simulink model "control_pos_no_lineal"  (R2020a)
settings: Solver=VariableStepAuto  StartTime=0.0  StopTime=5  RelTol=1e-3
values from neighbouring files (symbols this model uses):
  Kp = (2*pi*freq)^2*eye(2)    [init_control_cartesiano.m]
  Kv = 2*sqrt(Kp)*eye(2)    [init_control_cartesiano.m]
  Robot = Robot.perturb(0.8)    [init_control_cartesiano.m]
undefined symbols (not defined in the file or in its folder): coriolis
libraries: roblocks x16, simulink x2
settings Model: Creator=Gianfranco  LastModifiedBy=HP

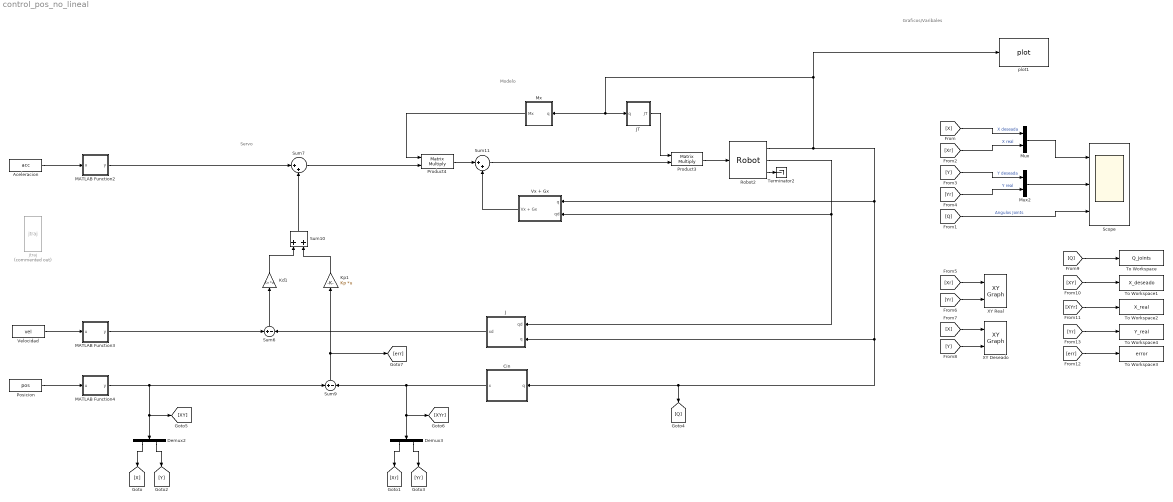
== system control_pos_no_lineal ==
  note: Graficos/Varibales
  note: Modelo
  note: Servo
  Aceleracion : FromWorkspace  VariableName=acc  SampleTime=-1  OutputAfterFinalValue=Holding final value
  Cin : Subsystem
  Demux2 : Demux  Outputs=2
  Demux3 : Demux  Outputs=2
  J : Subsystem
  JT : Subsystem
  Kd1 : Gain  Gain=Kv  Multiplication=Matrix(K*u)  SaturateOnIntegerOverflow=on  OutDataTypeStr=Inherit: Same as input  ParamDataTypeStr=Inherit: Same as input
  Kp1 : Gain  Gain=Kp  Multiplication=Matrix(K*u)  SaturateOnIntegerOverflow=on  OutDataTypeStr=Inherit: Same as input  ParamDataTypeStr=Inherit: Same as input
  MATLAB Function2 : MATLAB Function  TreatAsAtomicUnit=on
  MATLAB Function3 : MATLAB Function  TreatAsAtomicUnit=on
  MATLAB Function4 : MATLAB Function  TreatAsAtomicUnit=on
  Mux : Mux  Inputs=2
  Mux2 : Mux  Inputs=2
  Mx : Subsystem
  Posicion : FromWorkspace  VariableName=pos  SampleTime=-1  OutputAfterFinalValue=Holding final value
  Product3 : Product  Multiplication=Matrix(*)
  Product4 : Product  Multiplication=Matrix(*)
  Robot2 : roblocks/Arm/Robot  robot=Robot  q0=q0
      link override Integrator: InitialCondition=0
  Scope : Scope  NumInputPorts=3
  Sum10 : Sum  SaturateOnIntegerOverflow=on
  Sum11 : Sum  Inputs=|++  InputSameDT=on  SaturateOnIntegerOverflow=on  OutDataTypeStr=Inherit: Same as first input
  Sum6 : Sum  Inputs=+|-  InputSameDT=on  SaturateOnIntegerOverflow=on  OutDataTypeStr=Inherit: Same as first input
  Sum7 : Sum  Inputs=|++  InputSameDT=on  SaturateOnIntegerOverflow=on  OutDataTypeStr=Inherit: Same as first input
  Sum9 : Sum  Inputs=+|-  InputSameDT=on  SaturateOnIntegerOverflow=on  OutDataTypeStr=Inherit: Same as first input
  Terminator2 : Terminator
  To Workspace : ToWorkspace  VariableName=Q_joints  SaveFormat=Timeseries  SampleTime=-1
  To Workspace1 : ToWorkspace  VariableName=X_deseado  SaveFormat=Timeseries  SampleTime=-1
  To Workspace2 : ToWorkspace  VariableName=X_real  SaveFormat=Timeseries  SampleTime=-1
  To Workspace3 : ToWorkspace  VariableName=error  SaveFormat=Timeseries  SampleTime=-1
  To Workspace4 : ToWorkspace  VariableName=Y_real  SaveFormat=Timeseries  SampleTime=-1
  Velocidad : FromWorkspace  VariableName=vel  SampleTime=-1  OutputAfterFinalValue=Holding final value
  Vx + Gx : Subsystem
  XY Deseado : simulink/Sinks/XY Graph  xmin=-2  xmax=2  ymin=-2  ymax=2  st=-1
  XY Real : simulink/Sinks/XY Graph  xmin=-2  xmax=2  ymin=-2  ymax=2  st=-1
  jtraj : roblocks/Toolbox/jtraj  Commented=on  q0=[0 0 0 0 0 0]  qf=[pi/4 pi/2 -pi/2 0 0 0]  tmax=10  ts=0.02
  plot1 : roblocks/Arm/plot  robot=Robot  fps=30  holdplot=on
  wires:
  Posicion/1 -> MATLAB Function4/1(u)
  Product3/1 -> Robot2/1
  Sum7/1 -> Product4/2
  Sum6/1 -> Kd1/1
  Sum9/1 -> [err], Kp1/1
  Product4/1 -> Sum11/1
  Aceleracion/1 -> MATLAB Function2/1(u)
  Velocidad/1 -> MATLAB Function3/1(u)
  Kd1/1 -> Sum10/1
  Robot2/3 -> Terminator2/1
  Kp1/1 -> Sum10/2
  Sum10/1 -> Sum7/2
  Mx/1(Mx) -> Product4/1
  Sum11/1 -> Product3/2
  JT/1(JT) -> Product3/1
  Robot2/2 -> Vx + Gx/2(qd), J/1(qd)
  Robot2/1 -> [Q], Cin/1(q), J/2(q), Vx + Gx/1(q), JT/1(q), Mx/1(q), plot1/1
  MATLAB Function2/1(y) -> Sum7/1
  MATLAB Function3/1(y) -> Sum6/1
  Vx + Gx/1(Vx + Gx) -> Sum11/2
  J/1(xd) -> Sum6/2
  Mux/1 -> Scope/1
  Demux3/2 -> [Yr]
  Demux3/1 -> [Xr]
  [X] -> Mux/1  "X deseada"
  [Xr] -> Mux/2  "X real"
  [Y] -> Mux2/1  "Y deseada"
  [Yr] -> Mux2/2  "Y real"
  Mux2/1 -> Scope/2
  [Q] -> Scope/3  "Angulos Joints"
  [Xr] -> XY Real/1
  [Yr] -> XY Real/2
  [Y] -> XY Deseado/2
  [X] -> XY Deseado/1
  Cin/1(x) -> [XYr], Demux3/1, Sum9/2
  [XY] -> To Workspace1/1
  [Q] -> To Workspace/1
  [XYr] -> To Workspace2/1
  [err] -> To Workspace3/1
  Demux2/1 -> [X]
  Demux2/2 -> [Y]
  MATLAB Function4/1(y) -> Sum9/1, Demux2/1, [XY]
  [Yr] -> To Workspace4/1

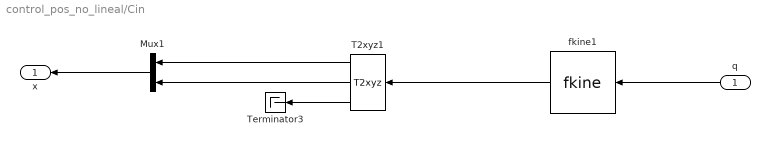
== system control_pos_no_lineal/Cin ==
  q : Inport
  Mux1 : Mux  Inputs=2
  T2xyz1 : roblocks/Toolbox/T2xyz
  Terminator3 : Terminator
  fkine1 : roblocks/Arm/fkine  robot=Robot
  x : Outport
  wires:
  T2xyz1/3 -> Terminator3/1
  fkine1/1 -> T2xyz1/1
  Mux1/1 -> x/1
  T2xyz1/2 -> Mux1/2
  T2xyz1/1 -> Mux1/1
  q/1 -> fkine1/1

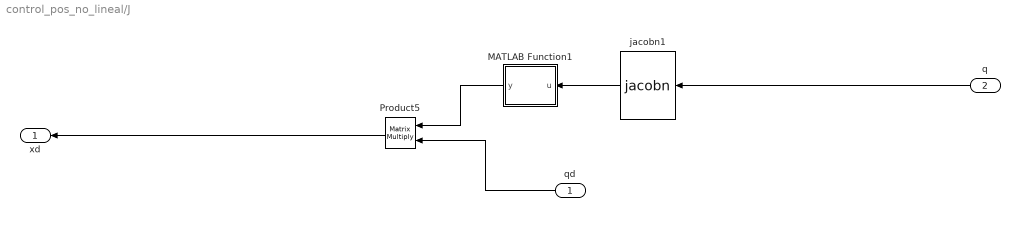
== system control_pos_no_lineal/J ==
  qd : Inport
  q : Inport  Port=2
  MATLAB Function1 : MATLAB Function  TreatAsAtomicUnit=on
  Product5 : Product  Multiplication=Matrix(*)
  jacobn1 : roblocks/Arm/jacobn  robot=Robot
  xd : Outport
  wires:
  jacobn1/1 -> MATLAB Function1/1(u)
  Product5/1 -> xd/1
  MATLAB Function1/1(y) -> Product5/1
  qd/1 -> Product5/2
  q/1 -> jacobn1/1

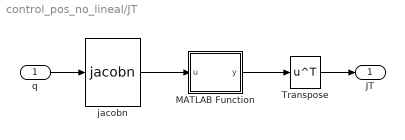
== system control_pos_no_lineal/JT ==
  q : Inport
  MATLAB Function : MATLAB Function  TreatAsAtomicUnit=on
  Transpose : Math  Operator=transpose  SaturateOnIntegerOverflow=on
  jacobn : roblocks/Arm/jacobn  robot=Robot
  JT : Outport
  wires:
  q/1 -> jacobn/1
  jacobn/1 -> MATLAB Function/1(u)
  Transpose/1 -> JT/1
  MATLAB Function/1(y) -> Transpose/1

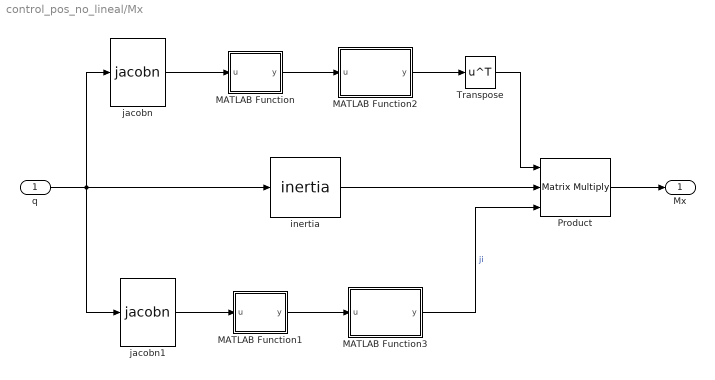
== system control_pos_no_lineal/Mx ==
  q : Inport
  MATLAB Function : MATLAB Function  TreatAsAtomicUnit=on
  MATLAB Function1 : MATLAB Function  TreatAsAtomicUnit=on
  MATLAB Function2 : MATLAB Function  TreatAsAtomicUnit=on
  MATLAB Function3 : MATLAB Function  TreatAsAtomicUnit=on
  Product : Product  Inputs=3  Multiplication=Matrix(*)
  Transpose : Math  Operator=transpose  SaturateOnIntegerOverflow=on
  inertia : roblocks/Arm/inertia  robot=Robot
  jacobn : roblocks/Arm/jacobn  robot=Robot
  jacobn1 : roblocks/Arm/jacobn  robot=Robot
  Mx : Outport
  wires:
  q/1 -> jacobn1/1, inertia/1, jacobn/1
  jacobn1/1 -> MATLAB Function1/1(u)
  MATLAB Function1/1(y) -> MATLAB Function3/1(u)
  Product/1 -> Mx/1
  inertia/1 -> Product/2
  jacobn/1 -> MATLAB Function/1(u)
  Transpose/1 -> Product/1
  MATLAB Function/1(y) -> MATLAB Function2/1(u)
  MATLAB Function3/1(y) -> Product/3  "ji"
  MATLAB Function2/1(y) -> Transpose/1

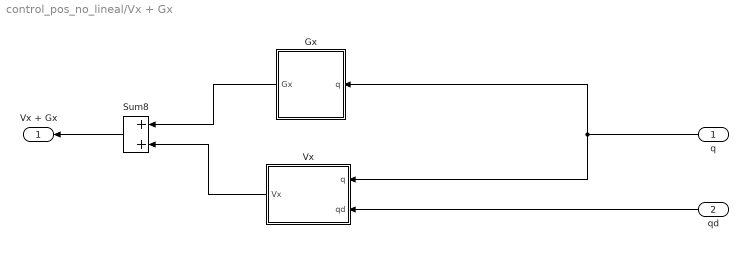
== system control_pos_no_lineal/Vx + Gx ==
  q : Inport
  qd : Inport  Port=2
  Gx : Subsystem
  Sum8 : Sum
  Vx : Subsystem
  Vx + Gx : Outport
  wires:
  Gx/1(Gx) -> Sum8/1
  Vx/1(Vx) -> Sum8/2
  Sum8/1 -> Vx + Gx/1
  qd/1 -> Vx/2(qd)
  q/1 -> Gx/1(q), Vx/1(q)

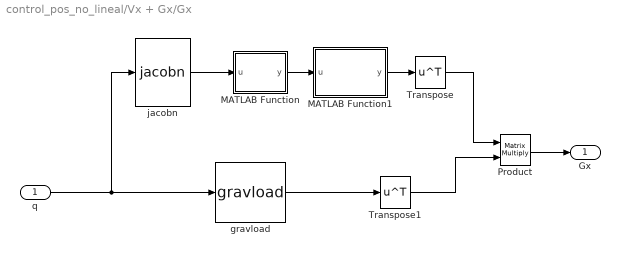
== system control_pos_no_lineal/Vx + Gx/Gx ==
  q : Inport
  MATLAB Function : MATLAB Function  TreatAsAtomicUnit=on
  MATLAB Function1 : MATLAB Function  TreatAsAtomicUnit=on
  Product : Product  Multiplication=Matrix(*)
  Transpose : Math  Operator=transpose  SaturateOnIntegerOverflow=on
  Transpose1 : Math  Operator=transpose  SaturateOnIntegerOverflow=on
  gravload : roblocks/Arm/gravload  robot=Robot
  jacobn : roblocks/Arm/jacobn  robot=Robot
  Gx : Outport
  wires:
  q/1 -> gravload/1, jacobn/1
  Product/1 -> Gx/1
  gravload/1 -> Transpose1/1
  jacobn/1 -> MATLAB Function/1(u)
  MATLAB Function/1(y) -> MATLAB Function1/1(u)
  Transpose1/1 -> Product/2
  MATLAB Function1/1(y) -> Transpose/1
  Transpose/1 -> Product/1

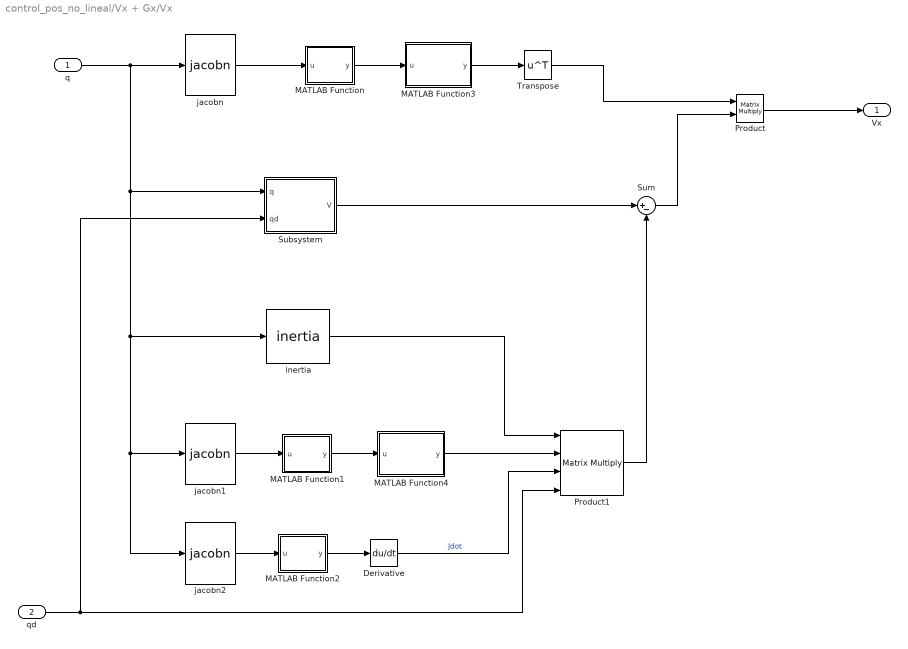
== system control_pos_no_lineal/Vx + Gx/Vx ==
  q : Inport
  qd : Inport  Port=2
  Derivative : Derivative
  MATLAB Function : MATLAB Function  TreatAsAtomicUnit=on
  MATLAB Function1 : MATLAB Function  TreatAsAtomicUnit=on
  MATLAB Function2 : MATLAB Function  TreatAsAtomicUnit=on
  MATLAB Function3 : MATLAB Function  TreatAsAtomicUnit=on
  MATLAB Function4 : MATLAB Function  TreatAsAtomicUnit=on
  Product : Product  Multiplication=Matrix(*)
  Product1 : Product  Inputs=4  Multiplication=Matrix(*)
  Subsystem : Subsystem
  Sum : Sum  Inputs=|+-
  Transpose : Math  Operator=transpose  SaturateOnIntegerOverflow=on
  inertia : roblocks/Arm/inertia  robot=Robot
  jacobn : roblocks/Arm/jacobn  robot=Robot
  jacobn1 : roblocks/Arm/jacobn  robot=Robot
  jacobn2 : roblocks/Arm/jacobn  robot=Robot
  Vx : Outport
  wires:
  MATLAB Function3/1(y) -> Transpose/1
  MATLAB Function/1(y) -> MATLAB Function3/1(u)
  jacobn/1 -> MATLAB Function/1(u)
  Sum/1 -> Product/2
  q/1 -> Subsystem/1(q), inertia/1, jacobn2/1, jacobn1/1, jacobn/1
  jacobn1/1 -> MATLAB Function1/1(u)
  MATLAB Function1/1(y) -> MATLAB Function4/1(u)
  jacobn2/1 -> MATLAB Function2/1(u)
  MATLAB Function2/1(y) -> Derivative/1
  inertia/1 -> Product1/1
  MATLAB Function4/1(y) -> Product1/2
  Derivative/1 -> Product1/3  "Jdot"
  qd/1 -> Subsystem/2(qd), Product1/4
  Product1/1 -> Sum/2
  Subsystem/1(V) -> Sum/1
  Transpose/1 -> Product/1
  Product/1 -> Vx/1

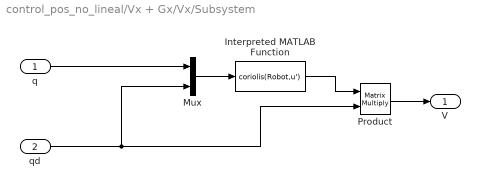
== system control_pos_no_lineal/Vx + Gx/Vx/Subsystem ==
  q : Inport
  qd : Inport  Port=2
  Interpreted MATLAB Function : MATLABFcn  MATLABFcn=coriolis(Robot,u')  OutputDimensions=[2,2]  Output1D=off
  Mux : Mux  Inputs=2
  Product : Product  Multiplication=Matrix(*)
  V : Outport
  wires:
  Product/1 -> V/1
  Interpreted MATLAB Function/1 -> Product/1
  Mux/1 -> Interpreted MATLAB Function/1
  q/1 -> Mux/1
  qd/1 -> Mux/2, Product/2

== matlab function control_pos_no_lineal/Vx + Gx/Vx/MATLAB Function3 ==
  data: u input; y output
function y = inversJac(u)

y = u^(-1);

== matlab function control_pos_no_lineal/Vx + Gx/Vx/MATLAB Function4 ==
  data: u input; y output
function y = inversJac(u)

y = u^(-1);

== matlab function control_pos_no_lineal/JT/MATLAB Function ==
  data: u input; y output
function y = reshape(u)

y = u(1:2,1:2);

== matlab function control_pos_no_lineal/MATLAB Function3 ==
  data: u input; y output
function y = reshape(u)

y = u(1:2,:);

== matlab function control_pos_no_lineal/MATLAB Function4 ==
  data: u input; y output
function y = reshape(u)

y = u(1:2,:);

== matlab function control_pos_no_lineal/Mx/MATLAB Function ==
  data: u input; y output
function y = reshape(u)

y = u(1:2,1:2);

== matlab function control_pos_no_lineal/Mx/MATLAB Function1 ==
  data: u input; y output
function y = reshape(u)

y = u(1:2,1:2);

== matlab function control_pos_no_lineal/Mx/MATLAB Function2 ==
  data: u input; y output
function y = inversJac(u)

y = u^(-1);

== matlab function control_pos_no_lineal/Mx/MATLAB Function3 ==
  data: u input; y output
function y = inversJac(u)

y = u^(-1);

== matlab function control_pos_no_lineal/Vx + Gx/Gx/MATLAB Function ==
  data: u input; y output
function y = reshape(u)

y = u(1:2,1:2);

== matlab function control_pos_no_lineal/MATLAB Function2 ==
  data: u input; y output
function y = reshape(u)

y = u(1:2,:);

== matlab function control_pos_no_lineal/Vx + Gx/Gx/MATLAB Function1 ==
  data: u input; y output
function y = inversJac(u)

y = u^(-1);

== matlab function control_pos_no_lineal/J/MATLAB Function1 ==
  data: u input; y output
function y = reshape(u)

y = u(1:2,1:2);

== matlab function control_pos_no_lineal/Vx + Gx/Vx/MATLAB Function ==
  data: u input; y output
function y = reshape(u)

y = u(1:2,1:2);

== matlab function control_pos_no_lineal/Vx + Gx/Vx/MATLAB Function1 ==
  data: u input; y output
function y = reshape(u)

y = u(1:2,1:2);

== matlab function control_pos_no_lineal/Vx + Gx/Vx/MATLAB Function2 ==
  data: u input; y output
function y = reshape(u)

y = u(1:2,1:2);
